simulink model "TiltCopter_TOSTO_v3"  (R2015a)
settings: Solver=ode45  StartTime=0.0  StopTime=10  RelTol=1e-3
values from neighbouring files (symbols this model uses):
  b = 0.55/2    (= 0.275)    [TiltCopter_Parameters_TOSTO_v3.m]
  B0 = 1.399e04    (= 13990)    [TiltCopter_Parameters_TOSTO_v3.m]
  B1 = 1150    [TiltCopter_Parameters_TOSTO_v3.m]
  B2 = 37.46    [TiltCopter_Parameters_TOSTO_v3.m]
  B3 = 1    [TiltCopter_Parameters_TOSTO_v3.m]
  degtorad = pi/180    (= 0.0174532925199)    [TiltCopter_Parameters_TOSTO_v3.m]
  dLMN = [dLdp  0    0 ... (first row only)    [TiltCopter_Parameters_TOSTO_v3.m]
  g = 9.81    [TiltCopter_Parameters_TOSTO_v3.m]
  I_Pi = diag([8.450e-5 8.450e-5 4.580e-5])    [TiltCopter_Parameters_TOSTO_v3.m]
  In = diag([Ixx Iyy Izz])    [TiltCopter_Parameters_TOSTO_v3.m]
  InInv = In\eye(3)    [TiltCopter_Parameters_TOSTO_v3.m]
  KaD = 5.4    [TiltCopter_Parameters_TOSTO_v3.m]
  KaI = 3.6    [TiltCopter_Parameters_TOSTO_v3.m]
  KaN = 38    [TiltCopter_Parameters_TOSTO_v3.m]
  KaP = 8.0    (= 8)    [TiltCopter_Parameters_TOSTO_v3.m]
  Kba = sqrt(KaD/KaI)    [TiltCopter_Parameters_TOSTO_v3.m]
  Kbp = sqrt(Kdp/Kip)    [TiltCopter_Parameters_TOSTO_v3.m]
  Kbq = sqrt(Kdq/Kiq)    [TiltCopter_Parameters_TOSTO_v3.m]
  Kbr = sqrt(Kdr/Kir)    [TiltCopter_Parameters_TOSTO_v3.m]
  Kdp = 0.0499    [TiltCopter_Parameters_TOSTO_v3.m]
  Kdq = 0.0499    [TiltCopter_Parameters_TOSTO_v3.m]
  Kdr = 0.0153    [TiltCopter_Parameters_TOSTO_v3.m]
  Kip = 0.304    [TiltCopter_Parameters_TOSTO_v3.m]
  Kiq = 0.304    [TiltCopter_Parameters_TOSTO_v3.m]
  Kir = 0.125    [TiltCopter_Parameters_TOSTO_v3.m]
  KPD = 0.00512    [TiltCopter_Parameters_TOSTO_v3.m]
  KPP = 1.61    [TiltCopter_Parameters_TOSTO_v3.m]
  Kpp = 0.298    [TiltCopter_Parameters_TOSTO_v3.m]
  Kpq = 0.298    [TiltCopter_Parameters_TOSTO_v3.m]
  Kpr = 0.135    [TiltCopter_Parameters_TOSTO_v3.m]
  Kq = Cq*ro*A*R^3    (= 2.88925724261e-07)    [TiltCopter_Parameters_TOSTO_v3.m]
  KRD = 0.00512    [TiltCopter_Parameters_TOSTO_v3.m]
  KRP = 1.61    [TiltCopter_Parameters_TOSTO_v3.m]
  Kt = Ct*ro*A*R^2    (= 2.46191978476e-05)    [TiltCopter_Parameters_TOSTO_v3.m]
  m = 1.510    (= 1.51)    [TiltCopter_Parameters_TOSTO_v3.m]
  m_servo = p(1)    [TiltCopter_Parameters_TOSTO_v3.m]
  Mb = diag([m m m])    [TiltCopter_Parameters_TOSTO_v3.m]
  MbInv = Mb\eye(3)    [TiltCopter_Parameters_TOSTO_v3.m]
  N = 1/Tf    (= 100)    [TiltCopter_Parameters_TOSTO_v3.m]
  omega_hover = OMEhov    [TiltCopter_Parameters_TOSTO_v3.m]
  pitchMax = pi/6    (= 0.523598775598)    [TiltCopter_Parameters_TOSTO_v3.m]
  q_servo = p(2)    [TiltCopter_Parameters_TOSTO_v3.m]
  rollMax = pi/6    (= 0.523598775598)    [TiltCopter_Parameters_TOSTO_v3.m]
  satp = 1.5    [TiltCopter_Parameters_TOSTO_v3.m]
  satq = 1.5    [TiltCopter_Parameters_TOSTO_v3.m]
  satr = 1    [TiltCopter_Parameters_TOSTO_v3.m]
  ServoMotor_Gain = 1.409e04    (= 14090)    [TiltCopter_Parameters_TOSTO_v3.m]
  tau = 0.055257    [TiltCopter_Parameters_TOSTO_v3.m]
  U = [-1; 0; 0; 0]    [Main_tiltCopter_TOSTO_v3.m]
  x1 = [m q]    [TiltCopter_Parameters_TOSTO_v3.m]
  yawRateMax = pi/2    (= 1.57079632679)    [TiltCopter_Parameters_TOSTO_v3.m]
undefined symbols (not defined in the file or in its folder): i, KPI, KRI
libraries: aerolibutil x10, simulink x6
(part 2 of 2)

== system TiltCopter_TOSTO_v3/TiltCopter/Actuators/Traslational Force_4 ==
  alpha_i : Inport
  omega_i : Inport  Port=2
  Product : Product  Multiplication=Matrix(*)
  R_BP4 : MATLAB Function  TreatAsAtomicUnit=on
  Thrust computation : Subsystem
  F_i : Outport
  wires:
  Thrust computation/1(Vector_Thrust_i) -> Product/2
  Product/1 -> F_i/1
  omega_i/1 -> Thrust computation/1(omega_i)
  R_BP4/1(Rotation_matrix) -> Product/1
  alpha_i/1 -> R_BP4/1(alpha_4)

== system TiltCopter_TOSTO_v3/TiltCopter/Actuators/Servo_Motor 1/Angle [rad] -> Pulse [ms] ==
  Pulse [ms] : Inport
  Add : Sum  Inputs=+-
  Constant : Constant  Value=q_servo
  Linear fitting gain : Gain  Gain=1/m_servo
  Angle [rad] : Outport
  wires:
  Constant/1 -> Add/2
  Add/1 -> Linear fitting gain/1
  Pulse [ms]/1 -> Add/1
  Linear fitting gain/1 -> Angle [rad]/1

== system TiltCopter_TOSTO_v3/TiltCopter/Actuators/Servo_Motor 2/Angle [rad] -> Pulse [ms] ==
  Pulse [ms] : Inport
  Add : Sum  Inputs=+-
  Constant : Constant  Value=q_servo
  Linear fitting gain : Gain  Gain=1/m_servo
  Angle [rad] : Outport
  wires:
  Constant/1 -> Add/2
  Add/1 -> Linear fitting gain/1
  Pulse [ms]/1 -> Add/1
  Linear fitting gain/1 -> Angle [rad]/1

== system TiltCopter_TOSTO_v3/TiltCopter/Actuators/Servo_Motor 3/Angle [rad] -> Pulse [ms] ==
  Pulse [ms] : Inport
  Add : Sum  Inputs=+-
  Constant : Constant  Value=q_servo
  Linear fitting gain : Gain  Gain=1/m_servo
  Angle [rad] : Outport
  wires:
  Constant/1 -> Add/2
  Add/1 -> Linear fitting gain/1
  Pulse [ms]/1 -> Add/1
  Linear fitting gain/1 -> Angle [rad]/1

== system TiltCopter_TOSTO_v3/TiltCopter/Actuators/Servo_Motor 4/Angle [rad] -> Pulse [ms] ==
  Pulse [ms] : Inport
  Add : Sum  Inputs=+-
  Constant : Constant  Value=q_servo
  Linear fitting gain : Gain  Gain=1/m_servo
  Angle [rad] : Outport
  wires:
  Constant/1 -> Add/2
  Add/1 -> Linear fitting gain/1
  Pulse [ms]/1 -> Add/1
  Linear fitting gain/1 -> Angle [rad]/1

== system TiltCopter_TOSTO_v3/TiltCopter/Actuators/Traslational Force_1/Thrust computation ==
  omega_i : Inport
  Constant : Constant  Value=-Kt
  Constant1 : Constant  Value=0
  Constant2 : Constant  Value=0
  Mux : Mux  Inputs=3
  Product : Product
  Product1 : Product
  Vector_Thrust_i : Outport
  wires:
  Constant2/1 -> Mux/2
  omega_i/1 -> Product/2, Product/1
  Product/1 -> Product1/1
  Constant1/1 -> Mux/1
  Mux/1 -> Vector_Thrust_i/1
  Product1/1 -> Mux/3
  Constant/1 -> Product1/2

== system TiltCopter_TOSTO_v3/TiltCopter/Actuators/Traslational Force_2/Thrust computation ==
  omega_i : Inport
  Constant : Constant  Value=-Kt
  Constant1 : Constant  Value=0
  Constant2 : Constant  Value=0
  Mux : Mux  Inputs=3
  Product : Product
  Product1 : Product
  Vector_Thrust_i : Outport
  wires:
  Constant2/1 -> Mux/2
  omega_i/1 -> Product/2, Product/1
  Product/1 -> Product1/1
  Constant1/1 -> Mux/1
  Mux/1 -> Vector_Thrust_i/1
  Product1/1 -> Mux/3
  Constant/1 -> Product1/2

== system TiltCopter_TOSTO_v3/TiltCopter/Actuators/Traslational Force_3/Thrust computation ==
  omega_i : Inport
  Constant : Constant  Value=-Kt
  Constant1 : Constant  Value=0
  Constant2 : Constant  Value=0
  Mux : Mux  Inputs=3
  Product : Product
  Product1 : Product
  Vector_Thrust_i : Outport
  wires:
  Constant2/1 -> Mux/2
  omega_i/1 -> Product/2, Product/1
  Product/1 -> Product1/1
  Constant1/1 -> Mux/1
  Mux/1 -> Vector_Thrust_i/1
  Product1/1 -> Mux/3
  Constant/1 -> Product1/2

== system TiltCopter_TOSTO_v3/TiltCopter/Actuators/Traslational Force_4/Thrust computation ==
  omega_i : Inport
  Constant : Constant  Value=-Kt
  Constant1 : Constant  Value=0
  Constant2 : Constant  Value=0
  Mux : Mux  Inputs=3
  Product : Product
  Product1 : Product
  Vector_Thrust_i : Outport
  wires:
  Constant2/1 -> Mux/2
  omega_i/1 -> Product/2, Product/1
  Product/1 -> Product1/1
  Constant1/1 -> Mux/1
  Mux/1 -> Vector_Thrust_i/1
  Product1/1 -> Mux/3
  Constant/1 -> Product1/2

== matlab function TiltCopter_TOSTO_v3/TiltCopter/To body from Earth ==
  data: Alpha_e input; Earth input; body output
 function body = Tbe(Alpha_e, Earth)
%#codegen
phi = Alpha_e(1);
theta = Alpha_e(2);
psi = Alpha_e(3);

Sphi = sin(phi);
Cphi = cos(phi);
Stheta = sin(theta);
Ctheta = cos(theta);
Spsi = sin(psi);
Cpsi = cos(psi);

TBE = [        Ctheta*Cpsi               Ctheta*Spsi          -Stheta    ;
       Sphi*Stheta*Cpsi-Cphi*Spsi Sphi*Stheta*Spsi+Cphi*Cpsi Sphi*Ctheta ;
       Cphi*Stheta*Cpsi+Sphi*Spsi Cphi*Stheta*Spsi-Sphi*Cpsi Cphi*Ctheta];

body = TBE* Earth;

== matlab function TiltCopter_TOSTO_v3/TiltCopter/To Earth from body ==
  data: Alpha_e input; Earth output; body input
 function Earth = Tbet(Alpha_e, body)
%#codegen
phi = Alpha_e(1);
theta = Alpha_e(2);
psi = Alpha_e(3);

Sphi = sin(phi);
Cphi = cos(phi);
Stheta = sin(theta);
Ctheta = cos(theta);
Spsi = sin(psi);
Cpsi = cos(psi);

TBE = [        Ctheta*Cpsi               Ctheta*Spsi          -Stheta    ;
       Sphi*Stheta*Cpsi-Cphi*Spsi Sphi*Stheta*Spsi+Cphi*Cpsi Sphi*Ctheta ;
       Cphi*Stheta*Cpsi+Sphi*Spsi Cphi*Stheta*Spsi-Sphi*Cpsi Cphi*Ctheta];
TEB = TBE';

Earth = TEB* body;

== matlab function TiltCopter_TOSTO_v3/TiltCopter/To Earth from body_rates ==
  data: Alpha_e input; Rates_B input; Rates_E output
 function Rates_E = Einv(Alpha_e, Rates_B)
%#codegen
phi = Alpha_e(1);
theta = Alpha_e(2);

Sphi = sin(phi);
Cphi = cos(phi);
Ctheta = cos(theta);
Ttheta = tan(theta);

Einv = [1   Sphi*Ttheta    Cphi*Ttheta ;
        0       Cphi          -Sphi    ;
        0   Sphi/Ctheta    Cphi/Ctheta];

Rates_E = Einv* Rates_B;

== matlab function TiltCopter_TOSTO_v3/TiltCopter/Actuators/Traslational Force_1/R_BP1 ==
  data: Rotation_matrix output; alpha_1 input
function Rotation_matrix = fcn(alpha_1)
%#codegen

% Rotation matrix from group propeller 1 to body
R_BP1 = [ 1,0,0; 0, cos(alpha_1), -sin(alpha_1);0, sin(alpha_1),cos(alpha_1)];
      



Rotation_matrix = R_BP1;

== matlab function TiltCopter_TOSTO_v3/Mixer Function/NONLINEAR mixer/Inverted NONLINEAR mixer matrix ==
  data: Fx input; Fy input; T input; L input; M input; N input; y output; omega_hover parameter; Kt parameter; Kq parameter; b parameter
function y = fcn(Fx,Fy,T,L,M,N,omega_hover,Kt,Kq,b)
%#codegen

omega_1 = omega_hover;
omega_2 = omega_hover;
omega_3 = omega_hover;
omega_4 = omega_hover;

% Calcolo prima gli alpha per ottenere la Fx e Fy desiderata considerando
% una omega di hovering
alpha_2 = -asin(Fx/(Kt*(omega_2^2 + omega_4^2)));

alpha_1 = asin(Fy/(Kt*(omega_1^2 + omega_3^2)));
alpha_3 = -alpha_1;
alpha_4 = -alpha_2;

% A questo punto risolvo la matrice K_mix, considerando gli angoli noti e
% risolvo solo per omega_i
K_mix = [
    -Kt*cos(alpha_1),                      -Kt*cos(alpha_2),                    -Kt*cos(alpha_3),                    -Kt*cos(alpha_4);
                                   0, - Kq*sin(alpha_2) - Kt*b*cos(alpha_2),                                   0, Kq*sin(alpha_4) + Kt*b*cos(alpha_4);
 Kt*b*cos(alpha_1) - Kq*sin(alpha_1),                                     0, Kq*sin(alpha_3) - Kt*b*cos(alpha_3),                                   0;
 Kq*cos(alpha_1) + Kt*b*sin(alpha_1),   Kt*b*sin(alpha_2) - Kq*cos(alpha_2), Kq*cos(alpha_3) + Kt*b*sin(alpha_3), Kt*b*sin(alpha_4) - Kq*cos(alpha_4)];

Omega_result = inv(K_mix)*[T;L;M;N];
y = [Omega_result;alpha_1;alpha_2;alpha_3;alpha_4];

== matlab function TiltCopter_TOSTO_v3/Controllers/Attitude Controller/To body from Earth_rates ==
  data: Alpha_e input; Rates_B output; Rates_E input
 function Rates_B = E(Alpha_e, Rates_E)
%#codegen
phi = Alpha_e(1);       % Roll
theta = Alpha_e(2);     % Pitch
psi = Alpha_e(3);       % Yaw

E = [cos(psi)*cos(theta),cos(theta)*sin(psi),-sin(theta);
 cos(psi)*sin(phi)*sin(theta) - cos(phi)*sin(psi), cos(phi)*cos(psi) + sin(phi)*sin(psi)*sin(theta), cos(theta)*sin(phi);
 sin(phi)*sin(psi) + cos(phi)*cos(psi)*sin(theta), cos(phi)*sin(psi)*sin(theta) - cos(psi)*sin(phi), cos(phi)*cos(theta)];

Rates_B = E* Rates_E;

== matlab function TiltCopter_TOSTO_v3/Mixer Function/NONLINEAR mixer/round1 ==
  data: u input; y output
function y = fcn(u)
%#codegen
 risultato = round(u*100)/100;
y = risultato;

== matlab function TiltCopter_TOSTO_v3/Mixer Function/NONLINEAR mixer/round2 ==
  data: u input; y output
function y = fcn(u)
%#codegen
 risultato = round(u*100)/100;
y = risultato;

== matlab function TiltCopter_TOSTO_v3/Mixer Function/NONLINEAR mixer/round3 ==
  data: u input; y output
function y = fcn(u)
%#codegen
 risultato = round(u*100)/100;
y = risultato;

== matlab function TiltCopter_TOSTO_v3/Mixer Function/NONLINEAR mixer/round4 ==
  data: u input; y output
function y = fcn(u)
%#codegen
 risultato = round(u*100)/100;
y = risultato;

== matlab function TiltCopter_TOSTO_v3/TiltCopter/Actuators/Rotor-hub_1/Origin ==
  data: i input; b input; OBPi output
function OBPi = R_zi(i, b)
%#codegen
psi = (1-i)*pi/2;
Spsi = sin(psi);
Cpsi = cos(psi);

Rz = [ Cpsi Spsi 0 ;
      -Spsi Cpsi 0 ; 
        0    0   1];
    
RBPi = Rz;

OBPi = RBPi * b;

== matlab function TiltCopter_TOSTO_v3/TiltCopter/Actuators/Rotor-hub_1/To body from propeller ==
  data: Alpha input; i input; Propeller input; body output
 function body = RBPi(Alpha, i, Propeller)
%#codegen
Salpha = sin(Alpha);
Calpha = cos(Alpha);

psi = (1-i)*pi/2;
Spsi = sin(psi);
Cpsi = cos(psi);

Rx = [1     0      0   ; 
      0  Calpha Salpha ; 
      0 -Salpha Calpha]; 
Rz = [ Cpsi Spsi 0 ;
      -Spsi Cpsi 0 ; 
        0    0   1];
    
RBPi = Rz*Rx;

body = RBPi * Propeller;

== matlab function TiltCopter_TOSTO_v3/TiltCopter/Actuators/Rotor-hub_1/To body from propeller  ==
  data: Alpha input; i input; Propeller input; body output
 function body = RBPi(Alpha, i, Propeller)
%#codegen
Salpha = sin(Alpha);
Calpha = cos(Alpha);

psi = (1-i)*pi/2;
Spsi = sin(psi);
Cpsi = cos(psi);

Rx = [1     0      0   ; 
      0  Calpha Salpha ; 
      0 -Salpha Calpha]; 
Rz = [ Cpsi Spsi 0 ;
      -Spsi Cpsi 0 ; 
        0    0   1];
    
RBPi = Rz*Rx;

body = RBPi * Propeller;

== matlab function TiltCopter_TOSTO_v3/TiltCopter/Actuators/Traslational Force_2/R_BP2 ==
  data: Rotation_matrix output; alpha_2 input
function Rotation_matrix = fcn(alpha_2)
%#codegen

% Rotation matrix from Propeller group 2 to body
R_BP2 =[ 0, -cos(alpha_2), sin(alpha_2); 1,0,0; 0,sin(alpha_2),cos(alpha_2)];

Rotation_matrix =R_BP2;

== matlab function TiltCopter_TOSTO_v3/TiltCopter/Actuators/Traslational Force_3/R_BP3 ==
  data: Rotation_matrix output; alpha_3 input
function Rotation_matrix = fcn(alpha_3)
%#codegen

R_BP3 = [ -1, 0, 0;0, -cos(alpha_3), sin(alpha_3);0,  sin(alpha_3), cos(alpha_3)];

Rotation_matrix = R_BP3;

== matlab function TiltCopter_TOSTO_v3/TiltCopter/Actuators/Traslational Force_4/R_BP4 ==
  data: Rotation_matrix output; alpha_4 input
function Rotation_matrix = fcn(alpha_4)
%#codegen

R_BP4 = [0, cos(alpha_4), -sin(alpha_4); -1, 0, 0; 0, sin(alpha_4), cos(alpha_4)];

Rotation_matrix = R_BP4;

== matlab function TiltCopter_TOSTO_v3/TiltCopter/Actuators/Rotor-hub_1/To propeller from body ==
  data: Alpha input; i input; Propeller output; body input
 function Propeller = RPiB(Alpha, i, body)
%#codegen
Salpha = sin(Alpha);
Calpha = cos(Alpha);

psi = (1-i)*pi/2;
Spsi = sin(psi);
Cpsi = cos(psi);

Rx = [1     0      0   ; 
      0  Calpha Salpha ; 
      0 -Salpha Calpha]; 
Rz = [ Cpsi Spsi 0 ;
      -Spsi Cpsi 0 ; 
        0    0   1];
    
RBPi = Rz*Rx;
RPiB = RBPi';

Propeller = RPiB * body;

== matlab function TiltCopter_TOSTO_v3/TiltCopter/Actuators/Rotor-hub_1/To propeller from body  ==
  data: Alpha input; i input; Propeller output; body input
 function Propeller = RPiB(Alpha, i, body)
%#codegen
Salpha = sin(Alpha);
Calpha = cos(Alpha);

psi = (1-i)*pi/2;
Spsi = sin(psi);
Cpsi = cos(psi);

Rx = [1     0      0   ; 
      0  Calpha Salpha ; 
      0 -Salpha Calpha]; 
Rz = [ Cpsi Spsi 0 ;
      -Spsi Cpsi 0 ; 
        0    0   1];
    
RBPi = Rz*Rx;
RPiB = RBPi';

Propeller = RPiB * body;

== matlab function TiltCopter_TOSTO_v3/TiltCopter/Actuators/Rotor-hub_1/To propeller from body_dot ==
  data: Alpha input; dAlpha input; i input; Propeller output; body input
 function Propeller = RPiB_dot(Alpha,dAlpha, i, body)
%#codegen
Salpha = sin(Alpha);
Calpha = cos(Alpha);

psi = (1-i)*pi/2;
Spsi = sin(psi);
Cpsi = cos(psi);

Rx = [1     0      0   ; 
      0  Calpha Salpha ; 
      0 -Salpha Calpha]; 
Rxdot = dAlpha*[0     0       0   ; 
                0 -Salpha  Calpha ; 
                0 -Calpha -Salpha];  
  
Rz = [ Cpsi Spsi 0 ;
      -Spsi Cpsi 0 ; 
        0    0   1];
    
RBPidot = Rz*Rxdot;
RPiBdot = RBPidot'

Propeller = RPiBdot* body;

== matlab function TiltCopter_TOSTO_v3/TiltCopter/Actuators/Rotor-hub_2/Origin ==
  data: i input; b input; OBPi output
function OBPi = R_zi(i, b)
%#codegen
psi = (1-i)*pi/2;
Spsi = sin(psi);
Cpsi = cos(psi);

Rz = [ Cpsi Spsi 0 ;
      -Spsi Cpsi 0 ; 
        0    0   1];
    
RBPi = Rz;

OBPi = RBPi * b;

== matlab function TiltCopter_TOSTO_v3/TiltCopter/Actuators/Rotor-hub_2/To body from propeller ==
  data: Alpha input; i input; Propeller input; body output
 function body = RBPi(Alpha, i, Propeller)
%#codegen
Salpha = sin(Alpha);
Calpha = cos(Alpha);

psi = (1-i)*pi/2;
Spsi = sin(psi);
Cpsi = cos(psi);

Rx = [1     0      0   ; 
      0  Calpha Salpha ; 
      0 -Salpha Calpha]; 
Rz = [ Cpsi Spsi 0 ;
      -Spsi Cpsi 0 ; 
        0    0   1];
    
RBPi = Rz*Rx;

body = RBPi * Propeller;

== matlab function TiltCopter_TOSTO_v3/TiltCopter/Actuators/Rotor-hub_2/To body from propeller  ==
  data: Alpha input; i input; Propeller input; body output
 function body = RBPi(Alpha, i, Propeller)
%#codegen
Salpha = sin(Alpha);
Calpha = cos(Alpha);

psi = (1-i)*pi/2;
Spsi = sin(psi);
Cpsi = cos(psi);

Rx = [1     0      0   ; 
      0  Calpha Salpha ; 
      0 -Salpha Calpha]; 
Rz = [ Cpsi Spsi 0 ;
      -Spsi Cpsi 0 ; 
        0    0   1];
    
RBPi = Rz*Rx;

body = RBPi * Propeller;

== matlab function TiltCopter_TOSTO_v3/TiltCopter/Actuators/Rotor-hub_2/To propeller from body ==
  data: Alpha input; i input; Propeller output; body input
 function Propeller = RPiB(Alpha, i, body)
%#codegen
Salpha = sin(Alpha);
Calpha = cos(Alpha);

psi = (1-i)*pi/2;
Spsi = sin(psi);
Cpsi = cos(psi);

Rx = [1     0      0   ; 
      0  Calpha Salpha ; 
      0 -Salpha Calpha]; 
Rz = [ Cpsi Spsi 0 ;
      -Spsi Cpsi 0 ; 
        0    0   1];
    
RBPi = Rz*Rx;
RPiB = RBPi';

Propeller = RPiB * body;

== matlab function TiltCopter_TOSTO_v3/TiltCopter/Actuators/Rotor-hub_2/To propeller from body  ==
  data: Alpha input; i input; Propeller output; body input
 function Propeller = RPiB(Alpha, i, body)
%#codegen
Salpha = sin(Alpha);
Calpha = cos(Alpha);

psi = (1-i)*pi/2;
Spsi = sin(psi);
Cpsi = cos(psi);

Rx = [1     0      0   ; 
      0  Calpha Salpha ; 
      0 -Salpha Calpha]; 
Rz = [ Cpsi Spsi 0 ;
      -Spsi Cpsi 0 ; 
        0    0   1];
    
RBPi = Rz*Rx;
RPiB = RBPi';

Propeller = RPiB * body;

== matlab function TiltCopter_TOSTO_v3/TiltCopter/Actuators/Rotor-hub_2/To propeller from body_dot ==
  data: Alpha input; dAlpha input; i input; Propeller output; body input
 function Propeller = RPiB_dot(Alpha,dAlpha, i, body)
%#codegen
Salpha = sin(Alpha);
Calpha = cos(Alpha);

psi = (1-i)*pi/2;
Spsi = sin(psi);
Cpsi = cos(psi);

Rx = [1     0      0   ; 
      0  Calpha Salpha ; 
      0 -Salpha Calpha]; 
Rxdot = dAlpha*[0     0       0   ; 
                0 -Salpha  Calpha ; 
                0 -Calpha -Salpha];  
  
Rz = [ Cpsi Spsi 0 ;
      -Spsi Cpsi 0 ; 
        0    0   1];
    
RBPidot = Rz*Rxdot;
RPiBdot = RBPidot'

Propeller = RPiBdot* body;

== matlab function TiltCopter_TOSTO_v3/TiltCopter/Actuators/Rotor-hub_3/Origin ==
  data: i input; b input; OBPi output
function OBPi = R_zi(i, b)
%#codegen
psi = (1-i)*pi/2;
Spsi = sin(psi);
Cpsi = cos(psi);

Rz = [ Cpsi Spsi 0 ;
      -Spsi Cpsi 0 ; 
        0    0   1];
    
RBPi = Rz;

OBPi = RBPi * b;

== matlab function TiltCopter_TOSTO_v3/TiltCopter/Actuators/Rotor-hub_3/To body from propeller ==
  data: Alpha input; i input; Propeller input; body output
 function body = RBPi(Alpha, i, Propeller)
%#codegen
Salpha = sin(Alpha);
Calpha = cos(Alpha);

psi = (1-i)*pi/2;
Spsi = sin(psi);
Cpsi = cos(psi);

Rx = [1     0      0   ; 
      0  Calpha Salpha ; 
      0 -Salpha Calpha]; 
Rz = [ Cpsi Spsi 0 ;
      -Spsi Cpsi 0 ; 
        0    0   1];
    
RBPi = Rz*Rx;

body = RBPi * Propeller;

== matlab function TiltCopter_TOSTO_v3/TiltCopter/Actuators/Rotor-hub_3/To body from propeller  ==
  data: Alpha input; i input; Propeller input; body output
 function body = RBPi(Alpha, i, Propeller)
%#codegen
Salpha = sin(Alpha);
Calpha = cos(Alpha);

psi = (1-i)*pi/2;
Spsi = sin(psi);
Cpsi = cos(psi);

Rx = [1     0      0   ; 
      0  Calpha Salpha ; 
      0 -Salpha Calpha]; 
Rz = [ Cpsi Spsi 0 ;
      -Spsi Cpsi 0 ; 
        0    0   1];
    
RBPi = Rz*Rx;

body = RBPi * Propeller;

== matlab function TiltCopter_TOSTO_v3/TiltCopter/Actuators/Rotor-hub_3/To propeller from body ==
  data: Alpha input; i input; Propeller output; body input
 function Propeller = RPiB(Alpha, i, body)
%#codegen
Salpha = sin(Alpha);
Calpha = cos(Alpha);

psi = (1-i)*pi/2;
Spsi = sin(psi);
Cpsi = cos(psi);

Rx = [1     0      0   ; 
      0  Calpha Salpha ; 
      0 -Salpha Calpha]; 
Rz = [ Cpsi Spsi 0 ;
      -Spsi Cpsi 0 ; 
        0    0   1];
    
RBPi = Rz*Rx;
RPiB = RBPi';

Propeller = RPiB * body;

== matlab function TiltCopter_TOSTO_v3/TiltCopter/Actuators/Rotor-hub_3/To propeller from body  ==
  data: Alpha input; i input; Propeller output; body input
 function Propeller = RPiB(Alpha, i, body)
%#codegen
Salpha = sin(Alpha);
Calpha = cos(Alpha);

psi = (1-i)*pi/2;
Spsi = sin(psi);
Cpsi = cos(psi);

Rx = [1     0      0   ; 
      0  Calpha Salpha ; 
      0 -Salpha Calpha]; 
Rz = [ Cpsi Spsi 0 ;
      -Spsi Cpsi 0 ; 
        0    0   1];
    
RBPi = Rz*Rx;
RPiB = RBPi';

Propeller = RPiB * body;

== matlab function TiltCopter_TOSTO_v3/TiltCopter/Actuators/Rotor-hub_3/To propeller from body_dot ==
  data: Alpha input; dAlpha input; i input; Propeller output; body input
 function Propeller = RPiB_dot(Alpha,dAlpha, i, body)
%#codegen
Salpha = sin(Alpha);
Calpha = cos(Alpha);

psi = (1-i)*pi/2;
Spsi = sin(psi);
Cpsi = cos(psi);

Rx = [1     0      0   ; 
      0  Calpha Salpha ; 
      0 -Salpha Calpha]; 
Rxdot = dAlpha*[0     0       0   ; 
                0 -Salpha  Calpha ; 
                0 -Calpha -Salpha];  
  
Rz = [ Cpsi Spsi 0 ;
      -Spsi Cpsi 0 ; 
        0    0   1];
    
RBPidot = Rz*Rxdot;
RPiBdot = RBPidot'

Propeller = RPiBdot* body;

== matlab function TiltCopter_TOSTO_v3/TiltCopter/Actuators/Rotor-hub_4/Origin ==
  data: i input; b input; OBPi output
function OBPi = R_zi(i, b)
%#codegen
psi = (1-i)*pi/2;
Spsi = sin(psi);
Cpsi = cos(psi);

Rz = [ Cpsi Spsi 0 ;
      -Spsi Cpsi 0 ; 
        0    0   1];
    
RBPi = Rz;

OBPi = RBPi * b;

== matlab function TiltCopter_TOSTO_v3/TiltCopter/Actuators/Rotor-hub_4/To body from propeller ==
  data: Alpha input; i input; Propeller input; body output
 function body = RBPi(Alpha, i, Propeller)
%#codegen
Salpha = sin(Alpha);
Calpha = cos(Alpha);

psi = (1-i)*pi/2;
Spsi = sin(psi);
Cpsi = cos(psi);

Rx = [1     0      0   ; 
      0  Calpha Salpha ; 
      0 -Salpha Calpha]; 
Rz = [ Cpsi Spsi 0 ;
      -Spsi Cpsi 0 ; 
        0    0   1];
    
RBPi = Rz*Rx;

body = RBPi * Propeller;

== matlab function TiltCopter_TOSTO_v3/TiltCopter/Actuators/Rotor-hub_4/To body from propeller  ==
  data: Alpha input; i input; Propeller input; body output
 function body = RBPi(Alpha, i, Propeller)
%#codegen
Salpha = sin(Alpha);
Calpha = cos(Alpha);

psi = (1-i)*pi/2;
Spsi = sin(psi);
Cpsi = cos(psi);

Rx = [1     0      0   ; 
      0  Calpha Salpha ; 
      0 -Salpha Calpha]; 
Rz = [ Cpsi Spsi 0 ;
      -Spsi Cpsi 0 ; 
        0    0   1];
    
RBPi = Rz*Rx;

body = RBPi * Propeller;

== matlab function TiltCopter_TOSTO_v3/TiltCopter/Actuators/Rotor-hub_4/To propeller from body ==
  data: Alpha input; i input; Propeller output; body input
 function Propeller = RPiB(Alpha, i, body)
%#codegen
Salpha = sin(Alpha);
Calpha = cos(Alpha);

psi = (1-i)*pi/2;
Spsi = sin(psi);
Cpsi = cos(psi);

Rx = [1     0      0   ; 
      0  Calpha Salpha ; 
      0 -Salpha Calpha]; 
Rz = [ Cpsi Spsi 0 ;
      -Spsi Cpsi 0 ; 
        0    0   1];
    
RBPi = Rz*Rx;
RPiB = RBPi';

Propeller = RPiB * body;

== matlab function TiltCopter_TOSTO_v3/TiltCopter/Actuators/Rotor-hub_4/To propeller from body  ==
  data: Alpha input; i input; Propeller output; body input
 function Propeller = RPiB(Alpha, i, body)
%#codegen
Salpha = sin(Alpha);
Calpha = cos(Alpha);

psi = (1-i)*pi/2;
Spsi = sin(psi);
Cpsi = cos(psi);

Rx = [1     0      0   ; 
      0  Calpha Salpha ; 
      0 -Salpha Calpha]; 
Rz = [ Cpsi Spsi 0 ;
      -Spsi Cpsi 0 ; 
        0    0   1];
    
RBPi = Rz*Rx;
RPiB = RBPi';

Propeller = RPiB * body;

== matlab function TiltCopter_TOSTO_v3/TiltCopter/Actuators/Rotor-hub_4/To propeller from body_dot ==
  data: Alpha input; dAlpha input; i input; Propeller output; body input
 function Propeller = RPiB_dot(Alpha,dAlpha, i, body)
%#codegen
Salpha = sin(Alpha);
Calpha = cos(Alpha);

psi = (1-i)*pi/2;
Spsi = sin(psi);
Cpsi = cos(psi);

Rx = [1     0      0   ; 
      0  Calpha Salpha ; 
      0 -Salpha Calpha]; 
Rxdot = dAlpha*[0     0       0   ; 
                0 -Salpha  Calpha ; 
                0 -Calpha -Salpha];  
  
Rz = [ Cpsi Spsi 0 ;
      -Spsi Cpsi 0 ; 
        0    0   1];
    
RBPidot = Rz*Rxdot;
RPiBdot = RBPidot'

Propeller = RPiBdot* body;
